simulink model "GPCA_Alarm"  (Simulink 8.7)
settings: Solver=VariableStepAuto  StartTime=0.0  StopTime=10.0  RelTol=1e-3
libraries: simulink x14
(part 3 of 3)

== stateflow chart Alarm  Sub-System ==
  state Alarms
    state CheckAlarm [parallel]
      settings: executionOrder=1
      state CancelAlarm [parallel]
        settings: executionOrder=1
        state ON
          entry:cancelAlarm = currentAlarm;
          writeLog(3);
          during:cancelAlarm = currentAlarm;
        state OFF
        (default) -> Alarms.CheckAlarm.CancelAlarm.OFF
        Alarms.CheckAlarm.CancelAlarm.OFF -> Alarms.CheckAlarm.CancelAlarm.ON : [currentAlarm > 0 && OP_CMD_IN_Notification_Cancel]
        Alarms.CheckAlarm.CancelAlarm.ON -> Alarms.CheckAlarm.CancelAlarm.OFF
      state setHighestAlarm [function]
        (default) -> (junction 91) : {ALARM_OUT_Highest_Level_Alarm=Max_Alarm_Level;}
      state Level4 [parallel]
        settings: executionOrder=2
        state IsEmptyReservoir [parallel]
          settings: executionOrder=1
          state No
          state Yes
          (default) -> Alarms.CheckAlarm.Level4.IsEmptyReservoir.No [order 2]
          (default) -> Alarms.CheckAlarm.Level4.IsEmptyReservoir.Yes [order 1] : [SYS_STAT_IN_In_Therapy && SYS_STAT_IN_Reservoir_Empty]
          Alarms.CheckAlarm.Level4.IsEmptyReservoir.No -> Alarms.CheckAlarm.Level4.IsEmptyReservoir.Yes : [SYS_STAT_IN_In_Therapy && SYS_STAT_IN_Reservoir_Empty]
          Alarms.CheckAlarm.Level4.IsEmptyReservoir.Yes -> Alarms.CheckAlarm.Level4.IsEmptyReservoir.No [order 2] : [cancelAlarm == 1 && !SYS_STAT_IN_Reservoir_Empty]
          Alarms.CheckAlarm.Level4.IsEmptyReservoir.Yes -> Alarms.CheckAlarm.Level4.IsEmptyReservoir.Yes [order 1] : [SYS_STAT_IN_In_Therapy && SYS_STAT_IN_Reservoir_Empty]
        state IsHardwareError [parallel]
          settings: executionOrder=2
          state Yes
          state No
          (default) -> Alarms.CheckAlarm.Level4.IsHardwareError.No [order 2]
          (default) -> Alarms.CheckAlarm.Level4.IsHardwareError.Yes [order 1] : [SENSOR_IN_Battery_Depleted || SENSOR_IN_RTC_Error || SENSOR_IN_CPU_Error || SENSOR_IN_Memory_Corrupted || SENSOR_IN_Pump_Too_Hot || SENSOR_IN_WatchDog_Interrupt_Detected]
          Alarms.CheckAlarm.Level4.IsHardwareError.No -> Alarms.CheckAlarm.Level4.IsHardwareError.Yes : [SENSOR_IN_Battery_Depleted || SENSOR_IN_RTC_Error || SENSOR_IN_CPU_Error || SENSOR_IN_Memory_Corrupted || SENSOR_IN_Pump_Too_Hot || SENSOR_IN_WatchDog_Interrupt_Detected]
          Alarms.CheckAlarm.Level4.IsHardwareError.Yes -> Alarms.CheckAlarm.Level4.IsHardwareError.No : [cancelAlarm ==2 &&  ! (SENSOR_IN_Battery_Depleted || SENSOR_IN_RTC_Error || SENSOR_IN_CPU_Error || SENSOR_IN_Memory_Corrupted || SENSOR_IN_Pump_Too_Hot || SENSOR_IN_WatchDog_Interrupt_Detected)]
        state IsEnviromentalError [parallel]
          settings: executionOrder=3
          state Yes
          state No
          (default) -> Alarms.CheckAlarm.Level4.IsEnviromentalError.Yes [order 1] : [SENSOR_IN_Temperature_Out_Of_Range || SENSOR_IN_Humidity_Out_Of_Range || SENSOR_IN_Air_Pressure_Out_Of_Range]
          (default) -> Alarms.CheckAlarm.Level4.IsEnviromentalError.No [order 2]
          Alarms.CheckAlarm.Level4.IsEnviromentalError.No -> Alarms.CheckAlarm.Level4.IsEnviromentalError.Yes : [SENSOR_IN_Temperature_Out_Of_Range || SENSOR_IN_Humidity_Out_Of_Range || SENSOR_IN_Air_Pressure_Out_Of_Range]
          Alarms.CheckAlarm.Level4.IsEnviromentalError.Yes -> Alarms.CheckAlarm.Level4.IsEnviromentalError.No : [cancelAlarm == 3 && !(SENSOR_IN_Temperature_Out_Of_Range || SENSOR_IN_Humidity_Out_Of_Range || SENSOR_IN_Air_Pressure_Out_Of_Range)]
      state Level3 [parallel]
        settings: executionOrder=3
        state IsOverInfusionFlowRate [parallel]
          entry:checkOverInfusionFlowRate();
          during:checkOverInfusionFlowRate();
          exit:checkOverInfusionFlowRate();
          settings: executionOrder=1
          state Yes
            entry:overInfusion=1;
            during:overInfusion=1;
          state Check
            entry:checkOverInfusionFlowRate();
            during:checkOverInfusionFlowRate();
            exit:checkOverInfusionFlowRate();
          state Monitor
            entry:checkOverInfusionFlowRate();
            during:checkOverInfusionFlowRate();
            exit:checkOverInfusionFlowRate();
          state checkOverInfusionFlowRate [function]
            (default) -> (junction 116) : {overInfusion=0;}
            (junction 116) -> (junction 118) : [SYS_STAT_IN_In_Therapy]
            (junction 118) -> (junction 117) [order 1] : [SENSOR_IN_Flow_Rate_Monitored > DB_IN_Flow_Rate_High]{overInfusion=1;}
            (junction 118) -> (junction 119) [order 2] : [SENSOR_IN_Flow_Rate_Monitored > (IM_IN_Flow_Rate_Commanded  * ((100 + CONST_IN_Tolerance_Max)/100))]{overInfusion=1;}
            (junction 118) -> (junction 120) [order 3] : [SENSOR_IN_Flow_Rate_Monitored > (IM_IN_Flow_Rate_Commanded * ((100 + CONST_IN_Tolerance_Min) /100))]{overInfusion=2;}
          (default) -> Alarms.CheckAlarm.Level3.IsOverInfusionFlowRate.Check [order 3]
          (default) -> Alarms.CheckAlarm.Level3.IsOverInfusionFlowRate.Yes [order 1] : [overInfusion==1]
          Alarms.CheckAlarm.Level3.IsOverInfusionFlowRate.Yes -> Alarms.CheckAlarm.Level3.IsOverInfusionFlowRate.Yes [order 1] : [overInfusion==1]
          Alarms.CheckAlarm.Level3.IsOverInfusionFlowRate.Check -> Alarms.CheckAlarm.Level3.IsOverInfusionFlowRate.Yes [order 1] : [overInfusion==1]
          Alarms.CheckAlarm.Level3.IsOverInfusionFlowRate.Yes -> Alarms.CheckAlarm.Level3.IsOverInfusionFlowRate.Check [order 2] : [cancelAlarm==4]
          Alarms.CheckAlarm.Level3.IsOverInfusionFlowRate.Monitor -> Alarms.CheckAlarm.Level3.IsOverInfusionFlowRate.Yes [order 1] : [overInfusion==1 || overInfusionTimer > Step_Scaling_Factor(CONST_IN_Max_Duration_Over_Infusion, step_size)]{overInfusionTimer=0;}
          Alarms.CheckAlarm.Level3.IsOverInfusionFlowRate.Monitor -> Alarms.CheckAlarm.Level3.IsOverInfusionFlowRate.Check [order 2] : [overInfusion==0]{overInfusionTimer=0;}
          Alarms.CheckAlarm.Level3.IsOverInfusionFlowRate.Check -> Alarms.CheckAlarm.Level3.IsOverInfusionFlowRate.Monitor [order 2] : [overInfusion == 2]{overInfusionTimer=0;}
          Alarms.CheckAlarm.Level3.IsOverInfusionFlowRate.Monitor -> Alarms.CheckAlarm.Level3.IsOverInfusionFlowRate.Monitor [order 3] : [overInfusion == 2 ]{overInfusionTimer++;}
          (default) -> Alarms.CheckAlarm.Level3.IsOverInfusionFlowRate.Monitor [order 2] : [overInfusion==2]
        state IsOverInfusionVTBI [parallel]
          settings: executionOrder=2
          state Yes
          state No
          (default) -> Alarms.CheckAlarm.Level3.IsOverInfusionVTBI.Yes [order 1] : [SYS_STAT_IN_In_Therapy && SYS_STAT_IN_Volume_Infused >DB_IN_VTBI_High]
          (default) -> Alarms.CheckAlarm.Level3.IsOverInfusionVTBI.No [order 2]
          Alarms.CheckAlarm.Level3.IsOverInfusionVTBI.Yes -> Alarms.CheckAlarm.Level3.IsOverInfusionVTBI.Yes [order 1] : [SYS_STAT_IN_In_Therapy &&  SYS_STAT_IN_Volume_Infused >DB_IN_VTBI_High]
          Alarms.CheckAlarm.Level3.IsOverInfusionVTBI.No -> Alarms.CheckAlarm.Level3.IsOverInfusionVTBI.Yes : [SYS_STAT_IN_In_Therapy &&  SYS_STAT_IN_Volume_Infused >DB_IN_VTBI_High]
          Alarms.CheckAlarm.Level3.IsOverInfusionVTBI.Yes -> Alarms.CheckAlarm.Level3.IsOverInfusionVTBI.No [order 2] : [cancelAlarm==5 ]
        state IsAirInLine [parallel]
          settings: executionOrder=3
          state Yes
          state No
          (default) -> Alarms.CheckAlarm.Level3.IsAirInLine.Yes [order 1] : [SENSOR_IN_Air_In_line]
          (default) -> Alarms.CheckAlarm.Level3.IsAirInLine.No [order 2]
          Alarms.CheckAlarm.Level3.IsAirInLine.No -> Alarms.CheckAlarm.Level3.IsAirInLine.Yes : [SENSOR_IN_Air_In_line]
          Alarms.CheckAlarm.Level3.IsAirInLine.Yes -> Alarms.CheckAlarm.Level3.IsAirInLine.No : [cancelAlarm ==6 && !SENSOR_IN_Air_In_line]
        state IsOcclusion [parallel]
          settings: executionOrder=4
          state Yes
          state No
          (default) -> Alarms.CheckAlarm.Level3.IsOcclusion.Yes [order 1] : [SENSOR_IN_Occlusion]
          (default) -> Alarms.CheckAlarm.Level3.IsOcclusion.No [order 2]
          Alarms.CheckAlarm.Level3.IsOcclusion.No -> Alarms.CheckAlarm.Level3.IsOcclusion.Yes : [SENSOR_IN_Occlusion]
          Alarms.CheckAlarm.Level3.IsOcclusion.Yes -> Alarms.CheckAlarm.Level3.IsOcclusion.No : [cancelAlarm ==7 && !SENSOR_IN_Occlusion ]
        state IsDoor_Open [parallel]
          settings: executionOrder=5
          state No
          state Yes
          (default) -> Alarms.CheckAlarm.Level3.IsDoor_Open.No [order 2]
          (default) -> Alarms.CheckAlarm.Level3.IsDoor_Open.Yes [order 1] : [SENSOR_IN_Door_Open]
          Alarms.CheckAlarm.Level3.IsDoor_Open.No -> Alarms.CheckAlarm.Level3.IsDoor_Open.Yes : [SENSOR_IN_Door_Open]
          Alarms.CheckAlarm.Level3.IsDoor_Open.Yes -> Alarms.CheckAlarm.Level3.IsDoor_Open.No : [cancelAlarm ==8 && !SENSOR_IN_Door_Open]
      state Level2 [parallel]
        settings: executionOrder=4
        state IsLowReservoir [parallel]
          settings: executionOrder=1
          state No
          state Yes
          (default) -> Alarms.CheckAlarm.Level2.IsLowReservoir.No [order 2]
          (default) -> Alarms.CheckAlarm.Level2.IsLowReservoir.Yes [order 1] : [SYS_STAT_IN_In_Therapy && SYS_STAT_IN_Reservoir_Volume < CONST_IN_Low_Reservoir]
          Alarms.CheckAlarm.Level2.IsLowReservoir.No -> Alarms.CheckAlarm.Level2.IsLowReservoir.Yes : [SYS_STAT_IN_In_Therapy && SYS_STAT_IN_Reservoir_Volume < CONST_IN_Low_Reservoir]
          Alarms.CheckAlarm.Level2.IsLowReservoir.Yes -> Alarms.CheckAlarm.Level2.IsLowReservoir.No : [cancelAlarm ==9 && !(SYS_STAT_IN_Reservoir_Volume < CONST_IN_Low_Reservoir)]
      state Level1 [parallel]
        settings: executionOrder=5
        state IsUnderInfusion [parallel]
          entry: checkUnderInfusion();
          during:checkUnderInfusion();
          exit:checkUnderInfusion();
          settings: executionOrder=1
          state Yes
            entry:underInfusion=1;
            during:underInfusion=1;
          state Check
            entry: underInfusion=0;
            during:underInfusion=0;
          state Monitor
            entry:underInfusion=2;checkUnderInfusion();
            during:checkUnderInfusion();
          state checkUnderInfusion [function]
            (default) -> (junction 156) : {underInfusion=0;}
            (junction 156) -> (junction 157) : [SYS_STAT_IN_In_Therapy]
            (junction 157) -> (junction 158) [order 1] : [SENSOR_IN_Flow_Rate_Monitored < DB_IN_Flow_Rate_Low]{underInfusion=1;}
            (junction 157) -> (junction 159) [order 2] : [SENSOR_IN_Flow_Rate_Monitored < IM_IN_Flow_Rate_Commanded - (IM_IN_Flow_Rate_Commanded * (CONST_IN_Tolerance_Max/100))]{underInfusion=1;}
            (junction 157) -> (junction 160) [order 3] : [SENSOR_IN_Flow_Rate_Monitored < IM_IN_Flow_Rate_Commanded - (IM_IN_Flow_Rate_Commanded * (CONST_IN_Tolerance_Min/100))]{underInfusion=2;}
          (default) -> Alarms.CheckAlarm.Level1.IsUnderInfusion.Yes [order 1] : [underInfusion==1]
          (default) -> Alarms.CheckAlarm.Level1.IsUnderInfusion.Check [order 3]
          Alarms.CheckAlarm.Level1.IsUnderInfusion.Check -> Alarms.CheckAlarm.Level1.IsUnderInfusion.Yes [order 1] : [underInfusion==1]
          Alarms.CheckAlarm.Level1.IsUnderInfusion.Yes -> Alarms.CheckAlarm.Level1.IsUnderInfusion.Check : [cancelAlarm==10]
          Alarms.CheckAlarm.Level1.IsUnderInfusion.Monitor -> Alarms.CheckAlarm.Level1.IsUnderInfusion.Yes [order 1] : [underInfusion==1 ||underInfusionTimer > Step_Scaling_Factor(CONST_IN_Max_Duration_Under_Infusion, step_size)] {underInfusionTimer=0;}
          Alarms.CheckAlarm.Level1.IsUnderInfusion.Monitor -> Alarms.CheckAlarm.Level1.IsUnderInfusion.Check [order 3] : [underInfusion==0]{underInfusionTimer=0.0;}
          Alarms.CheckAlarm.Level1.IsUnderInfusion.Check -> Alarms.CheckAlarm.Level1.IsUnderInfusion.Monitor [order 2] : [underInfusion==2]{underInfusionTimer=0.0;}
          (default) -> Alarms.CheckAlarm.Level1.IsUnderInfusion.Monitor [order 2] : [underInfusion==2]
          Alarms.CheckAlarm.Level1.IsUnderInfusion.Monitor -> Alarms.CheckAlarm.Level1.IsUnderInfusion.Monitor [order 2] : [underInfusion==2]{underInfusionTimer++;}
        state IsFlowRateNotStable [parallel]
          settings: executionOrder=2
          state Yes
          state No
          (default) -> Alarms.CheckAlarm.Level1.IsFlowRateNotStable.Yes [order 1] : [SYS_STAT_IN_In_Therapy && SENSOR_IN_Flow_Rate_Not_Stable]
          (default) -> Alarms.CheckAlarm.Level1.IsFlowRateNotStable.No [order 2]
          Alarms.CheckAlarm.Level1.IsFlowRateNotStable.No -> Alarms.CheckAlarm.Level1.IsFlowRateNotStable.Yes : [SYS_STAT_IN_In_Therapy && SENSOR_IN_Flow_Rate_Not_Stable]
          Alarms.CheckAlarm.Level1.IsFlowRateNotStable.Yes -> Alarms.CheckAlarm.Level1.IsFlowRateNotStable.No : [cancelAlarm==11 && !SENSOR_IN_Flow_Rate_Not_Stable]
        state IsPausedTimeExceeded [parallel]
          settings: executionOrder=4
          state counting
            entry: pausedtimer++;
            during: pausedtimer++;
            exit: pausedtimer++;
          state No
            entry:pausedtimer=0;
            during:pausedtimer=0;
            exit:pausedtimer=0;
          state Yes
          (default) -> Alarms.CheckAlarm.Level1.IsPausedTimeExceeded.counting [order 2] : [IM_IN_Current_System_Mode == 6 || IM_IN_Current_System_Mode == 7 ||  IM_IN_Current_System_Mode == 8 ]{pausedtimer=0;}
          (default) -> Alarms.CheckAlarm.Level1.IsPausedTimeExceeded.No [order 3]
          Alarms.CheckAlarm.Level1.IsPausedTimeExceeded.No -> Alarms.CheckAlarm.Level1.IsPausedTimeExceeded.counting [order 2] : [IM_IN_Current_System_Mode == 6 || IM_IN_Current_System_Mode == 7 ||  IM_IN_Current_System_Mode == 8 ]{pausedtimer=0;}
          Alarms.CheckAlarm.Level1.IsPausedTimeExceeded.Yes -> Alarms.CheckAlarm.Level1.IsPausedTimeExceeded.No : [cancelAlarm==13]
          Alarms.CheckAlarm.Level1.IsPausedTimeExceeded.No -> Alarms.CheckAlarm.Level1.IsPausedTimeExceeded.Yes [order 1] : [(IM_IN_Current_System_Mode == 6 || IM_IN_Current_System_Mode == 7 ||  IM_IN_Current_System_Mode == 8 ) &&  Step_Scaling_Factor(CONST_IN_Max_Paused_Duration,step_size) == 1.0]
          Alarms.CheckAlarm.Level1.IsPausedTimeExceeded.counting -> Alarms.CheckAlarm.Level1.IsPausedTimeExceeded.Yes : [ pausedtimer >= Step_Scaling_Factor(CONST_IN_Max_Paused_Duration,step_size)]
          (default) -> Alarms.CheckAlarm.Level1.IsPausedTimeExceeded.Yes [order 1] : [(IM_IN_Current_System_Mode == 6 || IM_IN_Current_System_Mode == 7 ||  IM_IN_Current_System_Mode == 8 ) &&  Step_Scaling_Factor(CONST_IN_Max_Paused_Duration,step_size) == 1.0]
        state IsIdleTimeExceeded [parallel]
          settings: executionOrder=3
          state counting
            entry: idletimer++;
            during: idletimer++;
            exit: idletimer++;
          state No
            entry:idletimer=0;
            during:idletimer=0;
            exit:idletimer=0;
          state Yes
          (default) -> Alarms.CheckAlarm.Level1.IsIdleTimeExceeded.counting [order 2] : [IM_IN_Current_System_Mode == 1]{idletimer=0;}
          (default) -> Alarms.CheckAlarm.Level1.IsIdleTimeExceeded.No [order 3]
          Alarms.CheckAlarm.Level1.IsIdleTimeExceeded.No -> Alarms.CheckAlarm.Level1.IsIdleTimeExceeded.counting [order 2] : [IM_IN_Current_System_Mode == 1]{idletimer=0;}
          Alarms.CheckAlarm.Level1.IsIdleTimeExceeded.No -> Alarms.CheckAlarm.Level1.IsIdleTimeExceeded.Yes [order 1] : [IM_IN_Current_System_Mode == 1 &&  Step_Scaling_Factor(CONST_IN_Max_Idle_Duration,step_size) == 1.0]
          Alarms.CheckAlarm.Level1.IsIdleTimeExceeded.Yes -> Alarms.CheckAlarm.Level1.IsIdleTimeExceeded.No : [cancelAlarm==12]
          Alarms.CheckAlarm.Level1.IsIdleTimeExceeded.counting -> Alarms.CheckAlarm.Level1.IsIdleTimeExceeded.Yes : [ idletimer >= Step_Scaling_Factor(CONST_IN_Max_Idle_Duration,step_size)]
          (default) -> Alarms.CheckAlarm.Level1.IsIdleTimeExceeded.Yes [order 1] : [IM_IN_Current_System_Mode == 1 &&  Step_Scaling_Factor(CONST_IN_Max_Idle_Duration,step_size) == 1.0]
        state IsConfigTimeWarning [parallel]
          settings: executionOrder=5
          state No
          state Yes
          (default) -> Alarms.CheckAlarm.Level1.IsConfigTimeWarning.No [order 2]
          (default) -> Alarms.CheckAlarm.Level1.IsConfigTimeWarning.Yes [order 1] : [CONFIG_IN_Config_Timer > Step_Scaling_Factor(CONST_IN_Config_Warning_Duration, step_size)]
          Alarms.CheckAlarm.Level1.IsConfigTimeWarning.No -> Alarms.CheckAlarm.Level1.IsConfigTimeWarning.Yes : [CONFIG_IN_Config_Timer > Step_Scaling_Factor(CONST_IN_Config_Warning_Duration, step_size)]
          Alarms.CheckAlarm.Level1.IsConfigTimeWarning.Yes -> Alarms.CheckAlarm.Level1.IsConfigTimeWarning.No : [cancelAlarm==14 && !(CONFIG_IN_Config_Timer > Step_Scaling_Factor(CONST_IN_Config_Warning_Duration, step_size))]
        state IsBatteryError [parallel]
          settings: executionOrder=6
          state Yes
          state No
          (default) -> Alarms.CheckAlarm.Level1.IsBatteryError.Yes [order 1] : [SENSOR_IN_Battery_Low || SENSOR_IN_Battery_Unable_To_Charge || SENSOR_IN_Supply_Voltage_Out_Of_Range]
          (default) -> Alarms.CheckAlarm.Level1.IsBatteryError.No [order 2]
          Alarms.CheckAlarm.Level1.IsBatteryError.No -> Alarms.CheckAlarm.Level1.IsBatteryError.Yes : [SENSOR_IN_Battery_Low || SENSOR_IN_Battery_Unable_To_Charge || SENSOR_IN_Supply_Voltage_Out_Of_Range]
          Alarms.CheckAlarm.Level1.IsBatteryError.Yes -> Alarms.CheckAlarm.Level1.IsBatteryError.No : [cancelAlarm==15 &&  !(SENSOR_IN_Battery_Low || SENSOR_IN_Battery_Unable_To_Charge || SENSOR_IN_Supply_Voltage_Out_Of_Range)]
        state IsPumpHot [parallel]
          settings: executionOrder=7
          state Yes
          state No
          (default) -> Alarms.CheckAlarm.Level1.IsPumpHot.Yes [order 1] : [SENSOR_IN_Pump_Overheated]
          (default) -> Alarms.CheckAlarm.Level1.IsPumpHot.No [order 2]
          Alarms.CheckAlarm.Level1.IsPumpHot.No -> Alarms.CheckAlarm.Level1.IsPumpHot.Yes : [SENSOR_IN_Pump_Overheated]
          Alarms.CheckAlarm.Level1.IsPumpHot.Yes -> Alarms.CheckAlarm.Level1.IsPumpHot.No : [cancelAlarm==16 && !SENSOR_IN_Pump_Overheated]
        state IsLoggingFailed [parallel]
          settings: executionOrder=8
          state Yes
          state No
          (default) -> Alarms.CheckAlarm.Level1.IsLoggingFailed.Yes [order 1] : [LOGGING_IN_Logging_Failed ]
          (default) -> Alarms.CheckAlarm.Level1.IsLoggingFailed.No [order 2]
          Alarms.CheckAlarm.Level1.IsLoggingFailed.No -> Alarms.CheckAlarm.Level1.IsLoggingFailed.Yes : [LOGGING_IN_Logging_Failed ]
          Alarms.CheckAlarm.Level1.IsLoggingFailed.Yes -> Alarms.CheckAlarm.Level1.IsLoggingFailed.No : [cancelAlarm==17 && !LOGGING_IN_Logging_Failed ]
        state IsSystemMonitorFailed [parallel]
          settings: executionOrder=9
          state Yes
          state No
          (default) -> Alarms.CheckAlarm.Level1.IsSystemMonitorFailed.Yes [order 1] : [SYS_MON_IN_System_Monitor_Failed]
          (default) -> Alarms.CheckAlarm.Level1.IsSystemMonitorFailed.No [order 2]
          Alarms.CheckAlarm.Level1.IsSystemMonitorFailed.No -> Alarms.CheckAlarm.Level1.IsSystemMonitorFailed.Yes : [SYS_MON_IN_System_Monitor_Failed]
          Alarms.CheckAlarm.Level1.IsSystemMonitorFailed.Yes -> Alarms.CheckAlarm.Level1.IsSystemMonitorFailed.No : [cancelAlarm==18 && !SYS_MON_IN_System_Monitor_Failed]
      state SetAlarmStatus [parallel]
        entry:setHighestAlarm();
        setCurrentAlarm();
        during:setHighestAlarm();
        setCurrentAlarm();
        exit:setHighestAlarm();
        setCurrentAlarm();
        cancelAlarm=0;
        settings: executionOrder=6
      state setCurrentAlarm [function]
        (default) -> (junction 240) : {currentAlarm = 0;Max_Alarm_Level=0;}
        (junction 240) -> (junction 241) [order 18] : [in(Alarms.CheckAlarm.Level1.IsSystemMonitorFailed.Yes)]{currentAlarm=18;Max_Alarm_Level=1;}
        (junction 240) -> (junction 241) [order 17] : [in(Alarms.CheckAlarm.Level1.IsLoggingFailed.Yes)]{currentAlarm=17;Max_Alarm_Level=1;}
        (junction 240) -> (junction 241) [order 16] : [in(Alarms.CheckAlarm.Level1.IsPumpHot.Yes)]{currentAlarm=16;Max_Alarm_Level=1;}
        (junction 240) -> (junction 241) [order 15] : [in(Alarms.CheckAlarm.Level1.IsBatteryError.Yes)]{currentAlarm=15;Max_Alarm_Level=1;}
        (junction 240) -> (junction 241) [order 14] : [in(Alarms.CheckAlarm.Level1.IsConfigTimeWarning.Yes)]{currentAlarm=14;Max_Alarm_Level=1;}
        (junction 240) -> (junction 241) [order 13] : [in(Alarms.CheckAlarm.Level1.IsPausedTimeExceeded.Yes)]{currentAlarm=13;Max_Alarm_Level=1;}
        (junction 240) -> (junction 241) [order 12] : [in(Alarms.CheckAlarm.Level1.IsIdleTimeExceeded.Yes)]{currentAlarm=12;Max_Alarm_Level=1;}
        (junction 240) -> (junction 241) [order 11] : [in(Alarms.CheckAlarm.Level1.IsFlowRateNotStable.Yes)]{currentAlarm=11;Max_Alarm_Level=1;}
        (junction 240) -> (junction 241) [order 1] : [in(Alarms.CheckAlarm.Level4.IsEmptyReservoir.Yes)]{currentAlarm=1;Max_Alarm_Level=4;}
        (junction 240) -> (junction 241) [order 2] : [in(Alarms.CheckAlarm.Level4.IsEnviromentalError.Yes)]{currentAlarm=2;Max_Alarm_Level=4;}
        (junction 240) -> (junction 241) [order 3] : [in(Alarms.CheckAlarm.Level4.IsHardwareError.Yes)]{currentAlarm=3;Max_Alarm_Level=4;}
        (junction 240) -> (junction 241) [order 10] : [in(Alarms.CheckAlarm.Level1.IsUnderInfusion.Yes)]{currentAlarm=10;Max_Alarm_Level=1;}
        (junction 240) -> (junction 241) [order 4] : [in(Alarms.CheckAlarm.Level3.IsOverInfusionFlowRate.Yes)]{currentAlarm=4;Max_Alarm_Level=3;}
        (junction 240) -> (junction 241) [order 5] : [in(Alarms.CheckAlarm.Level3.IsOverInfusionVTBI.Yes)]{currentAlarm=5;Max_Alarm_Level=3;}
        (junction 240) -> (junction 241) [order 9] : [in(Alarms.CheckAlarm.Level2.IsLowReservoir.Yes)] {currentAlarm=9;Max_Alarm_Level=2;}
        (junction 240) -> (junction 241) [order 6] : [in(Alarms.CheckAlarm.Level3.IsAirInLine.Yes)]{currentAlarm=6;Max_Alarm_Level=3;}
        (junction 240) -> (junction 241) [order 8] : [in(Alarms.CheckAlarm.Level3.IsDoor_Open.Yes)]{currentAlarm=8;Max_Alarm_Level=3;}
        (junction 240) -> (junction 241) [order 7] : [in(Alarms.CheckAlarm.Level3.IsOcclusion.Yes)]{currentAlarm=7;Max_Alarm_Level=3;}
    state Notification [parallel]
      settings: executionOrder=2
      state Visual [parallel]
        settings: executionOrder=1
        state OFF
          entry:ALARM_OUT_Visual_Notification_Message = 0;
          previousAlarm=0;
        state AlarmDisplay
          entry:ALARM_OUT_Visual_Notification_Message = currentAlarm;
          during:ALARM_OUT_Visual_Notification_Message = currentAlarm;
          exit:ALARM_OUT_Visual_Notification_Message = currentAlarm;
        (default) -> Alarms.Notification.Visual.OFF [order 2]
        (default) -> AlarmDisplay [order 1] : [currentAlarm > 0]
        Alarms.Notification.Visual.OFF -> AlarmDisplay : [currentAlarm > 0]
        AlarmDisplay -> Alarms.Notification.Visual.OFF [order 1] : [currentAlarm == 0]
        AlarmDisplay -> AlarmDisplay [order 2] : [currentAlarm > 0]
      state Audio [parallel]
        entry: ALARM_OUT_Is_Audio_Disabled=OP_CMD_IN_Disable_Audio;
        during: ALARM_OUT_Is_Audio_Disabled=OP_CMD_IN_Disable_Audio;
        exit: ALARM_OUT_Is_Audio_Disabled=OP_CMD_IN_Disable_Audio;
        settings: executionOrder=2
        state ON
          entry: ALARM_OUT_Audio_Notification_Command=CONST_IN_Audio_Level;
          during: ALARM_OUT_Audio_Notification_Command=CONST_IN_Audio_Level;
          exit: ALARM_OUT_Audio_Notification_Command=CONST_IN_Audio_Level;
        state OFF
          entry: ALARM_OUT_Audio_Notification_Command=0;
          during: ALARM_OUT_Audio_Notification_Command=0;
          exit: ALARM_OUT_Audio_Notification_Command=0;
        state Silenced
          entry: audioTimer = 0;ALARM_OUT_Audio_Notification_Command=0;audioTimer++;
          exit: ALARM_OUT_Audio_Notification_Command=0;
          during: audioTimer++;ALARM_OUT_Audio_Notification_Command=0;
        state Disabled
          entry: ALARM_OUT_Audio_Notification_Command=0;
          during: ALARM_OUT_Audio_Notification_Command=0;
          exit: ALARM_OUT_Audio_Notification_Command=0;
        (default) -> Alarms.Notification.Audio.OFF [order 4]
        Alarms.Notification.Audio.ON -> Alarms.Notification.Audio.ON [order 3] : [ALARM_OUT_Highest_Level_Alarm > 2 && OP_CMD_IN_Disable_Audio == 0]
        (default) -> Alarms.Notification.Audio.ON [order 3] : [ALARM_OUT_Highest_Level_Alarm > 2 && OP_CMD_IN_Disable_Audio == 0]
        Alarms.Notification.Audio.OFF -> Alarms.Notification.Audio.ON [order 3] : [ALARM_OUT_Highest_Level_Alarm > 2 && OP_CMD_IN_Disable_Audio == 0]
        Alarms.Notification.Audio.ON -> Alarms.Notification.Audio.OFF [order 4]
        (junction 210) -> Alarms.Notification.Audio.OFF
        Alarms.Notification.Audio.OFF -> (junction 209) [order 2]
        Alarms.Notification.Audio.OFF -> Disabled [order 1] : [OP_CMD_IN_Disable_Audio == 1]
        Alarms.Notification.Audio.ON -> Disabled [order 1] : [OP_CMD_IN_Disable_Audio == 1]
        Alarms.Notification.Audio.ON -> (junction 209) [order 2]
        (junction 211) -> Alarms.Notification.Audio.ON : [ALARM_OUT_Highest_Level_Alarm > 2 && OP_CMD_IN_Disable_Audio == 0]
        (junction 209) -> Silenced : [OP_CMD_IN_Disable_Audio == 2]
        Silenced -> (junction 210) [order 3] : [(audioTimer > Step_Scaling_Factor(CONST_IN_Audio_Auto_Enable_Duration,step_size)) || OP_CMD_IN_Disable_Audio == 0]
        Silenced -> (junction 211) [order 2]
        Disabled -> (junction 210) [order 3] : [OP_CMD_IN_Disable_Audio == 0]
        Disabled -> (junction 211) [order 2]
        Silenced -> Disabled [order 1] : [OP_CMD_IN_Disable_Audio == 1]
        (default) -> Silenced [order 2] : [OP_CMD_IN_Disable_Audio ==2]
        Disabled -> Silenced [order 1] : [OP_CMD_IN_Disable_Audio == 2]
        (default) -> Disabled [order 1] : [OP_CMD_IN_Disable_Audio ==1]
  note: step scaling factor returns the scaled time depending upon the step size.
      | If counter has to timeout after 100 seconds and if the step size is 0.1 second
      | the new timeout value = 100/0.1 = 1000 steps.
      | default will be one step = 1 second.
  state NOT_ON
  state writeLog(logEvent) [function]
    (default) -> (junction 233) : {ALARM_OUT_Log_Message_ID=logEvent;}
  state returnVal = Step_Scaling_Factor(inputVal,step_size) [function]
    (default) -> (junction 238) : {returnVal=inputVal/step_size;}
  (default) -> Alarms [order 1] : [TLM_MODE_IN_System_On]
  (default) -> NOT_ON [order 2]
  NOT_ON -> Alarms : [TLM_MODE_IN_System_On]
  Alarms -> NOT_ON : [!TLM_MODE_IN_System_On]
  data: logEvent function_input uint8; inputVal function_input double; returnVal function_output double; step_size function_input double; IM_IN_Flow_Rate_Commanded input uint8; IM_IN_Current_System_Mode input uint8; TLM_MODE_IN_System_On input boolean; SYS_MON_IN_System_Monitor_Failed input boolean; LOGGING_IN_Logging_Failed input boolean; OP_CMD_IN_Disable_Audio input uint8; OP_CMD_IN_Notification_Cancel input boolean; DB_IN_Flow_Rate_High input uint8; DB_IN_Flow_Rate_Low input uint8; DB_IN_VTBI_High input uint8; SENSOR_IN_Flow_Rate_Monitored input uint8; SENSOR_IN_Flow_Rate_Not_Stable input boolean; SENSOR_IN_Air_In_line input boolean; SENSOR_IN_Occlusion input boolean; SENSOR_IN_Door_Open input boolean; ALARM_OUT_Is_Audio_Disabled output uint8; ALARM_OUT_Visual_Notification_Message output uint8; ALARM_OUT_Audio_Notification_Command output uint8; overInfusion local uint8; overInfusionTimer local double; underInfusion local uint8; underInfusionTimer local double; ALARM_OUT_Highest_Level_Alarm output uint8; ALARM_OUT_Log_Message_ID output uint8; currentAlarm local uint8; previousAlarm local uint8; SENSOR_IN_Air_Pressure_Out_Of_Range input boolean; SENSOR_IN_Temperature_Out_Of_Range input boolean; SENSOR_IN_Humidity_Out_Of_Range input boolean; SENSOR_IN_Battery_Depleted input boolean; SENSOR_IN_Battery_Low input boolean; SENSOR_IN_Battery_Unable_To_Charge input boolean; SENSOR_IN_Supply_Voltage_Out_Of_Range input boolean; SENSOR_IN_CPU_Error input boolean; SENSOR_IN_RTC_Error input boolean; SENSOR_IN_WatchDog_Interrupt_Detected input boolean; SENSOR_IN_Memory_Corrupted input boolean; SENSOR_IN_Pump_Overheated input boolean; SENSOR_IN_Pump_Too_Hot input boolean; CONST_IN_Audio_Auto_Enable_Duration input double; CONST_IN_Audio_Level input uint8; CONST_IN_Low_Reservoir input uint8; CONST_IN_Max_Duration_Over_Infusion input double; CONST_IN_Max_Duration_Under_Infusion input double; CONST_IN_Tolerance_Max input uint8; CONST_IN_Tolerance_Min input uint8; CONST_IN_Config_Warning_Duration input double; CONST_IN_Max_Idle_Duration input double; CONST_IN_Max_Paused_Duration input double; audioTimer local double; cancelAlarm local uint8; SYS_STAT_IN_Reservoir_Empty input boolean; SYS_STAT_IN_Reservoir_Volume input uint8; SYS_STAT_IN_Volume_Infused input uint8; SYS_STAT_IN_In_Therapy input boolean; Max_Alarm_Level local uint8; CONFIG_IN_Config_Timer input double; idletimer local double; pausedtimer local double; step_size parameter double
